simulink model "Design2_20250221_2"  (R2024a)
settings: Solver=VariableStepAuto  StartTime=0.0  StopTime=1000  RelTol=1e-3
libraries: slpidlib x1
settings Model: Creator=ALCOT161  LastModifiedBy=ALCOT161

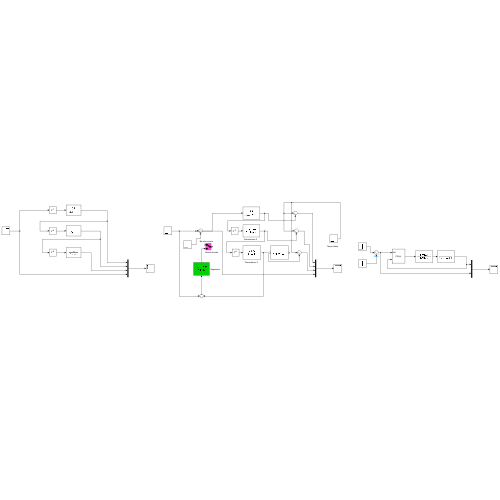
[thumbnail: Simulink's stored preview of the top-level diagram]
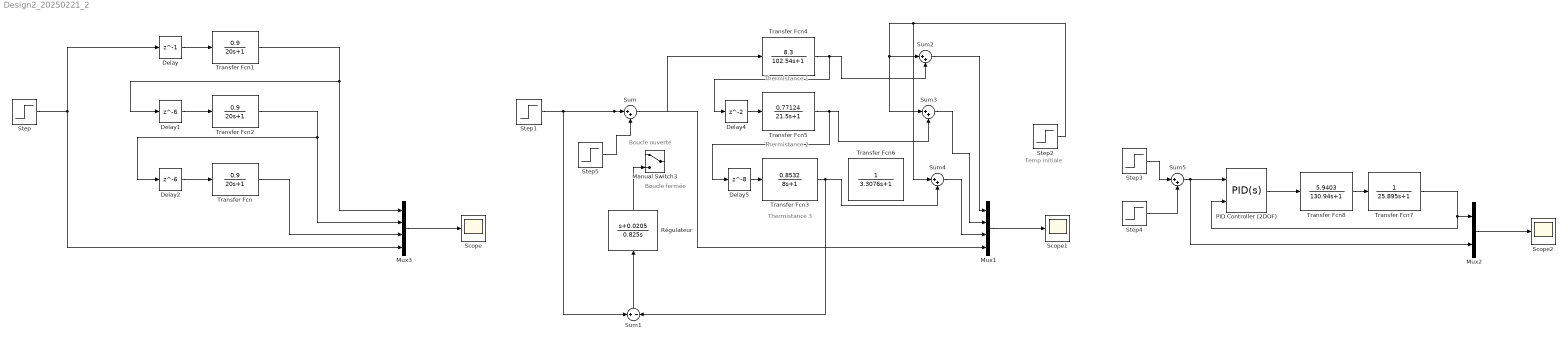
== system Design2_20250221_2 ==
  note: Thermistance 3
  note: Thermistance 2
  note: Thermistance 1
  note: Boucle fermée
  note: Boucle ouverte
  note: Temp initiale
  Delay : Delay  DelayLength=1  InitialCondition=0  SampleTime=1
  Delay1 : Delay  DelayLength=6  InitialCondition=0  SampleTime=1
  Delay2 : Delay  DelayLength=6  InitialCondition=0  SampleTime=1
  Delay4 : Delay  InitialCondition=0  SampleTime=1
  Delay5 : Delay  DelayLength=8  InitialCondition=0  SampleTime=1
  Manual Switch3 : ManualSwitch
  Mux1 : Mux
  Mux2 : Mux  Inputs=2
  Mux3 : Mux
  PID Controller (2DOF) : slpidlib/PID Controller (2DOF)  Controller=PID  Form=Parallel  TimeDomain=Continuous-time  UseExternalTs=off  SampleTime=-1  IntegratorMethod=Forward Euler  FilterMethod=Forward Euler  ControllerParametersSource=internal  P=3.74454447706948  I=0.0445535817708263  UseKiTs=off  D=51.4994682980153  UseExternalDerivativeSource=off  N=11.2712709683033  UseFilter=on  b=0.734946237693928  c=0.0139542516776796  TunerSelectOption=Transfer Function Based (PID Tuner App)  InitialConditionSource=internal  InitialConditionForIntegrator=0  InitialConditionForFilter=0  DifferentiatorICPrevScaledInput=0  ExternalReset=none  TrackingMode=off  Kt=1  LimitOutput=off  SatLimitsSource=internal  UpperSaturationLimit=inf  LowerSaturationLimit=-inf  LinearizeAsGain=on  AntiWindupMode=none  Kb=1  LimitIntegrator=off  UpperIntegratorSaturationLimit=inf  LowerIntegratorSaturationLimit=-inf  POutMin=[]  POutMax=[]  IOutMin=[]  IOutMax=[]  DOutMin=[]  DOutMax=[]  NOutMin=[]  NOutMax=[]  bOutMin=[]  bOutMax=[]  cOutMin=[]  cOutMax=[]  SumOutMin=[]  SumOutMax=[]  SaturationOutMin=[]  SaturationOutMax=[]  PParamMin=[]  PParamMax=[]  IParamMin=[]  IParamMax=[]  DParamMin=[]  DParamMax=[]  NParamMin=[]  NParamMax=[]  bParamMin=[]  bParamMax=[]  cParamMin=[]  cParamMax=[]  KbParamMin=[]  KbParamMax=[]  KtParamMin=[]  KtParamMax=[]  KbOutMin=[]  KbOutMax=[]  KtOutMin=[]  KtOutMax=[]  IntegratorOutMin=[]  IntegratorOutMax=[]  FilterOutMin=[]  FilterOutMax=[]  SumI1OutMin=[]  SumI1OutMax=[]  SumI2OutMin=[]  SumI2OutMax=[]  SumI3OutMin=[]  SumI3OutMax=[]  SumI4OutMin=[]  SumI4OutMax=[]  SumDOutMin=[]  SumDOutMax=[]  Sum1OutMin=[]  Sum1OutMax=[]  Sum2OutMin=[]  Sum2OutMax=[]  Sum3OutMin=[]  Sum3OutMax=[]  DifferentiatorOutMin=[]  DifferentiatorOutMax=[]  FilterDiffOutCoefMin=[]  FilterDiffOutCoefMax=[]  ReciprocalOutMin=[]  ReciprocalOutMax=[]  SumDenOutMin=[]  SumDenOutMax=[]  SumNumOutMin=[]  SumNumOutMax=[]  DivideOutMin=[]  DivideOutMax=[]  UdiffTsProdOutMin=[]  UdiffTsProdOutMax=[]  NTsProdOutMin=[]  NTsProdOutMax=[]  UintegralTsProdOutMin=[]  UintegralTsProdOutMax=[]  UngainTsProdOutMin=[]  UngainTsProdOutMax=[]  ClampingZeroOutDataTypeStr=Inherit: Inherit via back propagation  ClampingZeroOutMin=[]  ClampingZeroOutMax=[]  FilterDenConstantOutDataTypeStr=Inherit: Inherit via back propagation  FilterDenConstantOutMin=[]  FilterDenConstantOutMax=[]  PCopyOutDataTypeStr=Inherit: Inherit via back propagation  PCopyOutMin=[]  PCopyOutMax=[]  NCopyOutDataTypeStr=Inherit: Inherit via back propagation  NCopyOutMin=[]  NCopyOutMax=[]  IntegratorContinuousStateAttributes=''  IntegratorStateMustResolveToSignalObject=off  IntegratorRTWStateStorageClass=Auto  FilterContinuousStateAttributes=''  FilterStateMustResolveToSignalObject=off  FilterRTWStateStorageClass=Auto  ParallelPVariant=InternalParameters  IdealPVariant=Disabled  IVariant=InternalParameters  DVariant=InternalParameters  bVariant=InternalParameters  cVariant=InternalParameters  IntegratorVariant=Continuous  SatVariant=Disabled  AWVariant=Passthrough  PCopyVariant=Disabled  TRVariant=Disabled  FdbkBlocksVariant=Forward  IdealPFdbkVariant=Disabled  SatFdbkVariant=Disabled  DerivativeFilterVariant=ContFilter  NVariant=InternalParameters  NCopyVariant=Disabled  FilterICVariant=InternalICsFilter  IntegratorICVariant=InternalICs  ExternalResetVariant=Disabled  TRSumVariant=Passthrough  SumFdbkVariant=Disabled  SumVariant=Sum_PID  TsampFilterVariant=InternalTs  TsampNgainVariant=Passthrough  TsampIntegralVariant=Disabled_SignalSpec  ExternalSaturationOutDataTypeStr=Inherit: Same as second input  DerivativeSourceVariant=ErrorSignal
  Régulateur : TransferFcn  Numerator=[1 0.0205]  Denominator=[0.825 0]
  Scope : Scope
  Scope1 : Scope
  Scope2 : Scope
  Step : Step  Time=0  After=25  SampleTime=180
  Step1 : Step  Time=0  After=0.6  SampleTime=0
  Step2 : Step  Time=0  Before=24  After=24  SampleTime=180
  Step3 : Step  Time=0  Before=5  After=5  SampleTime=0
  Step4 : Step  Time=500  After=2  SampleTime=0
  Step5 : Step  Time=1000  After=0.2  SampleTime=0
  Sum{,2..5} (5 alike) : Sum  Inputs=|++
  Sum1 : Sum  Inputs=+|-  SampleTime=0
  Transfer Fcn : TransferFcn  Numerator=[0.9]  Denominator=[20 1]
  Transfer Fcn1 : TransferFcn  Numerator=[0.9]  Denominator=[20 1]
  Transfer Fcn2 : TransferFcn  Numerator=[0.9]  Denominator=[20 1]
  Transfer Fcn3 : TransferFcn  Numerator=[0.8532]  Denominator=[8 1]
  Transfer Fcn4 : TransferFcn  Numerator=[8.3]  Denominator=[102.54 1]
  Transfer Fcn5 : TransferFcn  Numerator=[0.77124]  Denominator=[21.5 1]
  Transfer Fcn6 : TransferFcn  Denominator=[3.3076 1]
  Transfer Fcn7 : TransferFcn  Denominator=[25.895 1]
  Transfer Fcn8 : TransferFcn  Numerator=[5.9403]  Denominator=[130.94 1]
  wires:
  Mux3/1 -> Scope/1
  Delay/1 -> Transfer Fcn1/1
  Delay1/1 -> Transfer Fcn2/1
  Delay2/1 -> Transfer Fcn/1
  Step/1 -> Mux3/4, Delay/1
  Transfer Fcn1/1 -> Delay1/1, Mux3/1
  Transfer Fcn2/1 -> Mux3/2, Delay2/1
  Transfer Fcn/1 -> Mux3/3
  Delay5/1 -> Transfer Fcn3/1
  Delay4/1 -> Transfer Fcn5/1
  Mux1/1 -> Scope1/1
  Sum1/1 -> Régulateur/1
  Sum/1 -> Transfer Fcn4/1
  Régulateur/1 -> Manual Switch3/2
  Step1/1 -> Mux1/4, Sum/1, Sum1/1
  Sum2/1 -> Mux1/1
  Sum3/1 -> Mux1/2
  Sum4/1 -> Mux1/3
  Step2/1 -> Sum3/1, Sum2/1, Sum4/1
  Transfer Fcn4/1 -> Delay4/1, Sum2/2
  Transfer Fcn3/1 -> Sum1/2, Sum4/2
  Transfer Fcn5/1 -> Delay5/1, Sum3/2
  Step5/1 -> Sum/2
  Mux2/1 -> Scope2/1
  PID Controller (2DOF)/1 -> Transfer Fcn8/1
  Transfer Fcn8/1 -> Transfer Fcn7/1
  Transfer Fcn7/1 -> Mux2/1, PID Controller (2DOF)/2
  Step3/1 -> Sum5/1
  Sum5/1 -> Mux2/2, PID Controller (2DOF)/1
  Step4/1 -> Sum5/2
